simulink subsystem "cascaded_pid_controller_cgn"  (R2025b)
settings: Solver=VariableStepAuto  StartTime=0.0  StopTime=10.0  RelTol=1e-3
undefined symbols (not defined in the file or in its folder): allow_PID_resets_flag, const_voltage, DiscIntNeverNeededParam, do_force_cmd_flag, do_moment_cmd_flag, dRb_error_inject, dRb_PID, dRb_sp_inject, dspblkCoreblockFVToolHelper, dt_control, dt_data, Eul_e_tol, eul_error_inject, eul_sp_inject, FF_maneuvers, FT_list_inject, gcbh, invFT_wrench, invMT_wrench, overwrite_FT_list_flag, overwrite_rate_error_flag, overwrite_rate_setpoint_flag, overwrite_state_error_flag, overwrite_state_setpoint_flag, qib_PID, quat_pid_integrator_limit, Rb_error_inject, Rb_PID, Rb_sp_inject, Ri_e_tol, RSFF_maneuvers, wb_error_inject, wb_PID, wb_sp_inject
libraries: slpidlib x3, simulink x1
settings Model: Creator=vulcangrip  LastModifiedBy=vulcangrip

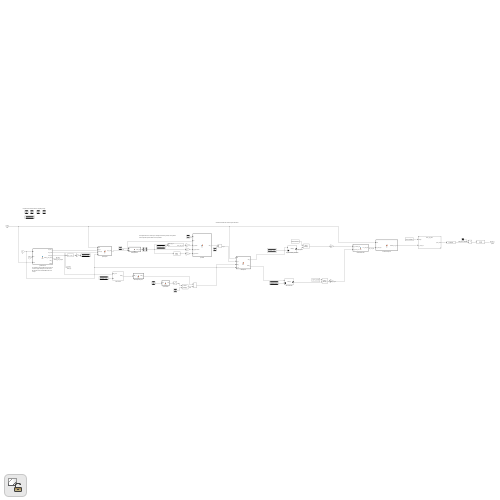
[thumbnail: Simulink's stored preview of the top-level diagram]
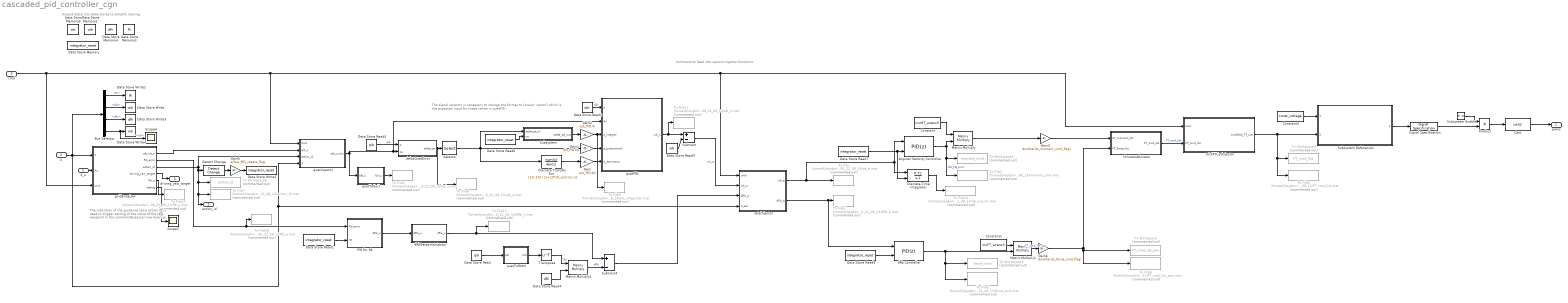
== system cascaded_pid_controller_cgn ==
  note: Unpack state into data-stores to simplify routing.
  note: Command to feed into various injector functions.
  note: The transition of the guidance law's action ID is used to trigger setting of the value of the idle waypoint in the commandExecuter one level up.
  note: The signal selector is necessary to change the format to [scalar; vector] which
      | is the expected input for these terms in quatPID.
  X_u : Inport  SampleTime=dt_control
  X : Inport  Port=2  SampleTime=dt_control
  cmd : Inport  Port=3  SampleTime=dt_control
  Subsystem Enable : EnablePort  PropagateVarSize=During execution  ShowOutputPort=on
  Angular Velocity Controller : slpidlib/PID Controller  Controller=PID  Form=Parallel  TimeDomain=Discrete-time  UseExternalTs=off  SampleTime=-1  IntegratorMethod=Forward Euler  FilterMethod=Forward Euler  ControllerParametersSource=internal  P=wb_PID.Kp  I=wb_PID.Ki  UseKiTs=off  D=wb_PID.Kd  UseExternalDerivativeSource=off  N=wb_PID.N  UseFilter=on  TunerSelectOption=Transfer Function Based (PID Tuner App)  InitialConditionSource=internal  InitialConditionForIntegrator=0  InitialConditionForFilter=0  DifferentiatorICPrevScaledInput=0  ExternalReset=rising  TrackingMode=off  Kt=1  LimitOutput=on  SatLimitsSource=internal  UpperSaturationLimit=wb_PID.output_sat  LowerSaturationLimit=-wb_PID.output_sat  LinearizeAsGain=on  AntiWindupMode=clamping  Kb=1  LimitIntegrator=on  UpperIntegratorSaturationLimit=wb_PID.int_sat  LowerIntegratorSaturationLimit=-wb_PID.int_sat  POutMin=[]  POutMax=[]  IOutMin=[]  IOutMax=[]  DOutMin=[]  DOutMax=[]  NOutMin=[]  NOutMax=[]  SumOutMin=[]  SumOutMax=[]  SaturationOutMin=[]  SaturationOutMax=[]  PParamMin=[]  PParamMax=[]  IParamMin=[]  IParamMax=[]  DParamMin=[]  DParamMax=[]  NParamMin=[]  NParamMax=[]  KbParamMin=[]  KbParamMax=[]  KtParamMin=[]  KtParamMax=[]  KbOutMin=[]  KbOutMax=[]  KtOutMin=[]  KtOutMax=[]  IntegratorOutMin=[]  IntegratorOutMax=[]  FilterOutMin=[]  FilterOutMax=[]  SumI1OutMin=[]  SumI1OutMax=[]  SumI2OutMin=[]  SumI2OutMax=[]  SumI3OutMin=[]  SumI3OutMax=[]  SumI4OutMin=[]  SumI4OutMax=[]  SumDOutMin=[]  SumDOutMax=[]  DifferentiatorOutMin=[]  DifferentiatorOutMax=[]  FilterDiffOutCoefMin=[]  FilterDiffOutCoefMax=[]  ReciprocalOutMin=[]  ReciprocalOutMax=[]  SumDenOutMin=[]  SumDenOutMax=[]  SumNumOutMin=[]  SumNumOutMax=[]  DivideOutMin=[]  DivideOutMax=[]  UdiffTsProdOutMin=[]  UdiffTsProdOutMax=[]  NTsProdOutMin=[]  NTsProdOutMax=[]  UintegralTsProdOutMin=[]  UintegralTsProdOutMax=[]  UngainTsProdOutMin=[]  UngainTsProdOutMax=[]  ClampingZeroOutDataTypeStr=Inherit: Inherit via back propagation  ClampingZeroOutMin=[]  ClampingZeroOutMax=[]  FilterDenConstantOutDataTypeStr=Inherit: Inherit via back propagation  FilterDenConstantOutMin=[]  FilterDenConstantOutMax=[]  PCopyOutDataTypeStr=Inherit: Inherit via back propagation  PCopyOutMin=[]  PCopyOutMax=[]  NCopyOutDataTypeStr=Inherit: Inherit via back propagation  NCopyOutMin=[]  NCopyOutMax=[]  IntegratorContinuousStateAttributes=''  IntegratorStateMustResolveToSignalObject=off  IntegratorRTWStateStorageClass=Auto  FilterContinuousStateAttributes=''  FilterStateMustResolveToSignalObject=off  FilterRTWStateStorageClass=Auto  ParallelPVariant=InternalParameters  IdealPVariant=Disabled  IVariant=InternalParameters  DVariant=InternalParameters  IntegratorVariant=Discrete  SatVariant=Enabled  AWVariant=DiscClampingParallel  PCopyVariant=Disabled  TRVariant=Disabled  FdbkBlocksVariant=Forward  IdealPFdbkVariant=Disabled  SatFdbkVariant=Disabled  DerivativeFilterVariant=ForwardEulerFilter  NVariant=InternalParameters  NCopyVariant=Disabled  FilterICVariant=InternalICsFilter  IntegratorICVariant=InternalICs  ExternalResetVariant=ExternalReset  TRSumVariant=Passthrough  SumFdbkVariant=Disabled  SumVariant=Sum_PID  TsampFilterVariant=InternalTs  TsampNgainVariant=Passthrough  TsampIntegralVariant=Disabled_SignalSpec  ExternalSaturationOutDataTypeStr=Inherit: Same as second input  DerivativeSourceVariant=ErrorSignal  PreIntVariant=InternalPreInt
  Bus Selector : BusSelector  OutputSignals=Ri,qib,dRi,wb
  Cast : DataTypeConversion  OutDataTypeStr=int32  SaturateOnIntegerOverflow=off  RndMeth=Floor
  Constant : Constant  Value=invMT_wrench
  Constant1 : Constant  Value=invFT_wrench
  Constant3 : Constant  Value=const_voltage
  Data Store Memory : DataStoreMemory  DataStoreName=integrator_reset  WriteAfterWriteMsg=warning  ShowAdditionalParam=off
  Data Store Memory2 : DataStoreMemory  DataStoreName=qib  WriteAfterWriteMsg=warning  InitialValue=[0 0 0 1]'  ShowAdditionalParam=off
  Data Store Memory3 : DataStoreMemory  DataStoreName=Ri  WriteAfterWriteMsg=warning  InitialValue=[0 0 0]'  ShowAdditionalParam=off
  Data Store Memory4 : DataStoreMemory  DataStoreName=dRi  WriteAfterWriteMsg=warning  InitialValue=[0 0 0]'  ShowAdditionalParam=off
  Data Store Memory5 : DataStoreMemory  DataStoreName=wb  WriteAfterWriteMsg=warning  InitialValue=[0 0 0]'  ShowAdditionalParam=off
  Data Store Read : DataStoreRead  DataStoreName=qib  IndexOptions=Index vector (dialog)  Indices=1  OutputSizes=1
  Data Store Read{1,6..7,9} (4 alike) : DataStoreRead  DataStoreName=integrator_reset  IndexOptions=Index vector (dialog)  Indices=1  OutputSizes=1
  Data Store Read2 : DataStoreRead  DataStoreName=qib  IndexOptions=Index vector (dialog)  Indices=1  OutputSizes=1
  Data Store Read3 : DataStoreRead  DataStoreName=wb  IndexOptions=Index vector (dialog)  Indices=1  OutputSizes=1
  Data Store Read4 : DataStoreRead  DataStoreName=dRi  IndexOptions=Index vector (dialog)  Indices=1  OutputSizes=1
  Data Store Read5 : DataStoreRead  DataStoreName=qib  IndexOptions=Index vector (dialog)  Indices=1  OutputSizes=1
  Data Store Write : DataStoreWrite  DataStoreName=qib  IndexOptions=Index vector (dialog)  Indices=1  OutputSizes=1
  Data Store Write1 : DataStoreWrite  DataStoreName=integrator_reset  IndexOptions=Index vector (dialog)  Indices=1  OutputSizes=1
  Data Store Write2 : DataStoreWrite  DataStoreName=Ri  IndexOptions=Index vector (dialog)  Indices=1  OutputSizes=1
  Data Store Write3 : DataStoreWrite  DataStoreName=dRi  IndexOptions=Index vector (dialog)  Indices=1  OutputSizes=1
  Data Store Write4 : DataStoreWrite  DataStoreName=wb  IndexOptions=Index vector (dialog)  Indices=1  OutputSizes=1
  Detect Change : simulink/Logic and Bit Operations/Detect Change  vinit=0  OutDataTypeStr=boolean
  Discrete Transfer Fcn : DiscreteTransferFcn  LoadFcn=dspblkCoreblockFVToolHelper(gcbh,'load');  Numerator=[10,-10]  Denominator=[1+10*dt_control,-1]
      settings: CopyFcn=dspblkCoreblockFVToolHelper(gcbh,'copy');  DeleteFcn=dspblkCoreblockFVToolHelper(gcbh,'close');  ModelCloseFcn=dspblkCoreblockFVToolHelper(gcbh,'close');  PreSaveFcn=dspblkCoreblockFVToolHelper(gcbh,'presave');  PostSaveFcn=dspblkCoreblockFVToolHelper(gcbh,'postsave');  CloseFcn=dspblkCoreblockFVToolHelper(gcbh,'close');
  Discrete-Time Integrator : DiscreteIntegrator  gainval=wb_PID.Ki  ExternalReset=rising  InitialCondition=[0;0;0]  SampleTime=dt_control  LimitOutput=on  UpperSaturationLimit=wb_PID.int_sat  LowerSaturationLimit=-wb_PID.int_sat  ICPrevOutput=DiscIntNeverNeededParam  ICPrevScaledInput=DiscIntNeverNeededParam
  Gain : Gain  Gain=qib_PID.Kd
  Gain1 : Gain  Gain=qib_PID.Kp
  Gain2 : Gain  Gain=qib_PID.Ki
  Gain3 : Gain  Gain=double(do_moment_cmd_flag)
  Gain4 : Gain  Gain=double(do_force_cmd_flag)
  Gain5 : Gain  Gain=allow_PID_resets_flag
  Matrix Multiply : Product  Multiplication=Matrix(*)
  Matrix Multiply1 : Product  Multiplication=Matrix(*)
  Matrix Multiply3 : Product  Multiplication=Matrix(*)
  PID for Rb : Subsystem
  Product : Product
  Scope1 : Scope
      settings: ActiveDisplayYMinimum=-1  ActiveDisplayYMaximum=1  DataLoggingVariableName=ScopeData3
  Scope4 : Scope
      settings: ActiveDisplayYMinimum=-1  ActiveDisplayYMaximum=1  DataLoggingVariableName=ScopeData6
  Selector : Selector  InputPortWidth=4  IndexOptions=Index vector (dialog)  Indices=[4 1 2 3]  OutputSizes=1
  Signal Specification : SignalSpecification  OutDataTypeStr=double
  Subsystem : Subsystem
  Subsystem Reference1 : Subsystem  ReferencedSubsystem=force_to_pwm
  Subtract : Sum  Inputs=+-
  Subtract4 : Sum  Inputs=+-
  To File : ToFile  Commented=on  Filename=/home/kjhaydon/Github/Robosub/SimulinkPlant/data/2026_07_06_22_08_13/wb_e.mat  MatrixName=wb_e  SaveFormat=Timeseries  SampleTime=dt_data
  To File1 : ToFile  Commented=on  Filename=/home/kjhaydon/Github/Robosub/SimulinkPlant/data/2026_07_06_22_08_13/dRb_e.mat  MatrixName=dRb_e  SaveFormat=Timeseries  SampleTime=dt_data
  To File10 : ToFile  Commented=on  Filename=/home/kjhaydon/Github/Robosub/SimulinkPlant/data/2026_07_06_22_08_13/Rb_e.mat  MatrixName=Rb_e  SaveFormat=Timeseries  SampleTime=dt_data
  To File11 : ToFile  Commented=on  Filename=/home/kjhaydon/Github/Robosub/SimulinkPlant/data/2026_07_06_22_08_13/wb_u.mat  MatrixName=wb_u  SaveFormat=Timeseries  SampleTime=dt_data
  To File12 : ToFile  Commented=on  Filename=/home/kjhaydon/Github/Robosub/SimulinkPlant/data/2026_07_06_22_08_13/dRb_u.mat  MatrixName=dRb_u  SaveFormat=Timeseries  SampleTime=dt_data
  To File13 : ToFile  Commented=on  Filename=/home/kjhaydon/Github/Robosub/SimulinkPlant/data/2026_07_06_22_08_13/Rb_u.mat  MatrixName=Rb_u  SaveFormat=Timeseries  SampleTime=dt_data
  To File14 : ToFile  Commented=on  Filename=/home/kjhaydon/Github/Robosub/SimulinkPlant/data/2026_07_06_22_08_13/wb_pid_int.mat  MatrixName=wb_pid_int  SaveFormat=Timeseries  SampleTime=dt_data
  To File2 : ToFile  Commented=on  Filename=/home/kjhaydon/Github/Robosub/SimulinkPlant/data/2026_07_06_22_08_13/moment_cmd.mat  MatrixName=moment_cmd  SaveFormat=Timeseries  SampleTime=dt_data
  To File3 : ToFile  Commented=on  Filename=/home/kjhaydon/Github/Robosub/SimulinkPlant/data/2026_07_06_22_08_13/Eul_u.mat  MatrixName=Eul_u  SaveFormat=Timeseries  SampleTime=dt_data
  To File4 : ToFile  Commented=on  Filename=/home/kjhaydon/Github/Robosub/SimulinkPlant/data/2026_07_06_22_08_13/FT_cmd_list.mat  MatrixName=FT_cmd_list  SaveFormat=Timeseries  SampleTime=dt_data
  To File5 : ToFile  Commented=on  Filename=/home/kjhaydon/Github/Robosub/SimulinkPlant/data/2026_07_06_22_08_13/force_cmd.mat  MatrixName=force_cmd  SaveFormat=Timeseries  SampleTime=dt_data
  To File6 : ToFile  Commented=on  Filename=/home/kjhaydon/Github/Robosub/SimulinkPlant/data/2026_07_06_22_08_13/FT_cmd_list_pos.mat  MatrixName=FT_cmd_list_pos  SaveFormat=Timeseries
  To File7 : ToFile  Commented=on  Filename=/home/kjhaydon/Github/Robosub/SimulinkPlant/data/2026_07_06_22_08_13/action_id.mat  MatrixName=action_id  SaveFormat=Timeseries  SampleTime=dt_control
  To File8 : ToFile  Commented=on  Filename=/home/kjhaydon/Github/Robosub/SimulinkPlant/data/2026_07_06_22_08_13/qib_e.mat  MatrixName=qib_e  SaveFormat=Timeseries  SampleTime=dt_data
  To File9 : ToFile  Commented=on  Filename=/home/kjhaydon/Github/Robosub/SimulinkPlant/data/2026_07_06_22_08_13/qib_integrator.mat  MatrixName=qib_integrator  SaveFormat=Timeseries  SampleTime=dt_data
  To Workspace : ToWorkspace  Commented=on  VariableName=FT_cmd_list_pos  SaveFormat=Timeseries  SampleTime=dt_data
  To Workspace2 : ToWorkspace  Commented=on  VariableName=FT_cmd_list  SaveFormat=Timeseries  SampleTime=dt_data
  To Workspace3 : ToWorkspace  Commented=on  VariableName=force_cmd  SaveFormat=Timeseries  SampleTime=dt_data
  To Workspace4 : ToWorkspace  Commented=on  VariableName=moment_cmd  SaveFormat=Timeseries  SampleTime=dt_data
  To Workspace5 : ToWorkspace  Commented=on  VariableName=action_id  SaveFormat=Timeseries  SampleTime=dt_control
  Transpose : Math  Operator=transpose
  dRb Controller : slpidlib/PID Controller  Controller=PID  Form=Parallel  TimeDomain=Discrete-time  UseExternalTs=off  SampleTime=-1  IntegratorMethod=Forward Euler  FilterMethod=Forward Euler  ControllerParametersSource=internal  P=dRb_PID.Kp  I=dRb_PID.Ki  UseKiTs=off  D=dRb_PID.Kd  UseExternalDerivativeSource=off  N=dRb_PID.N  UseFilter=on  TunerSelectOption=Transfer Function Based (PID Tuner App)  InitialConditionSource=internal  InitialConditionForIntegrator=0  InitialConditionForFilter=0  DifferentiatorICPrevScaledInput=0  ExternalReset=rising  TrackingMode=off  Kt=1  LimitOutput=on  SatLimitsSource=internal  UpperSaturationLimit=dRb_PID.output_sat  LowerSaturationLimit=-dRb_PID.output_sat  LinearizeAsGain=on  AntiWindupMode=clamping  Kb=1  LimitIntegrator=on  UpperIntegratorSaturationLimit=dRb_PID.int_sat  LowerIntegratorSaturationLimit=-dRb_PID.int_sat  POutMin=[]  POutMax=[]  IOutMin=[]  IOutMax=[]  DOutMin=[]  DOutMax=[]  NOutMin=[]  NOutMax=[]  SumOutMin=[]  SumOutMax=[]  SaturationOutMin=[]  SaturationOutMax=[]  PParamMin=[]  PParamMax=[]  IParamMin=[]  IParamMax=[]  DParamMin=[]  DParamMax=[]  NParamMin=[]  NParamMax=[]  KbParamMin=[]  KbParamMax=[]  KtParamMin=[]  KtParamMax=[]  KbOutMin=[]  KbOutMax=[]  KtOutMin=[]  KtOutMax=[]  IntegratorOutMin=[]  IntegratorOutMax=[]  FilterOutMin=[]  FilterOutMax=[]  SumI1OutMin=[]  SumI1OutMax=[]  SumI2OutMin=[]  SumI2OutMax=[]  SumI3OutMin=[]  SumI3OutMax=[]  SumI4OutMin=[]  SumI4OutMax=[]  SumDOutMin=[]  SumDOutMax=[]  DifferentiatorOutMin=[]  DifferentiatorOutMax=[]  FilterDiffOutCoefMin=[]  FilterDiffOutCoefMax=[]  ReciprocalOutMin=[]  ReciprocalOutMax=[]  SumDenOutMin=[]  SumDenOutMax=[]  SumNumOutMin=[]  SumNumOutMax=[]  DivideOutMin=[]  DivideOutMax=[]  UdiffTsProdOutMin=[]  UdiffTsProdOutMax=[]  NTsProdOutMin=[]  NTsProdOutMax=[]  UintegralTsProdOutMin=[]  UintegralTsProdOutMax=[]  UngainTsProdOutMin=[]  UngainTsProdOutMax=[]  ClampingZeroOutDataTypeStr=Inherit: Inherit via back propagation  ClampingZeroOutMin=[]  ClampingZeroOutMax=[]  FilterDenConstantOutDataTypeStr=Inherit: Inherit via back propagation  FilterDenConstantOutMin=[]  FilterDenConstantOutMax=[]  PCopyOutDataTypeStr=Inherit: Inherit via back propagation  PCopyOutMin=[]  PCopyOutMax=[]  NCopyOutDataTypeStr=Inherit: Inherit via back propagation  NCopyOutMin=[]  NCopyOutMax=[]  IntegratorContinuousStateAttributes=''  IntegratorStateMustResolveToSignalObject=off  IntegratorRTWStateStorageClass=Auto  FilterContinuousStateAttributes=''  FilterStateMustResolveToSignalObject=off  FilterRTWStateStorageClass=Auto  ParallelPVariant=InternalParameters  IdealPVariant=Disabled  IVariant=InternalParameters  DVariant=InternalParameters  IntegratorVariant=Discrete  SatVariant=Enabled  AWVariant=DiscClampingParallel  PCopyVariant=Disabled  TRVariant=Disabled  FdbkBlocksVariant=Forward  IdealPFdbkVariant=Disabled  SatFdbkVariant=Disabled  DerivativeFilterVariant=ForwardEulerFilter  NVariant=InternalParameters  NCopyVariant=Disabled  FilterICVariant=InternalICsFilter  IntegratorICVariant=InternalICs  ExternalResetVariant=ExternalReset  TRSumVariant=Passthrough  SumFdbkVariant=Disabled  SumVariant=Sum_PID  TsampFilterVariant=InternalTs  TsampNgainVariant=Passthrough  TsampIntegralVariant=Disabled_SignalSpec  ExternalSaturationOutDataTypeStr=Inherit: Same as second input  DerivativeSourceVariant=ErrorSignal  PreIntVariant=InternalPreInt
  dRbSetpointInjector : MATLAB Function  TreatAsAtomicUnit=on
  deltaQuatError : MATLAB Function  TreatAsAtomicUnit=on
  guidanceLaw : MATLAB Function  TreatAsAtomicUnit=on
  quatInjector : MATLAB Function  TreatAsAtomicUnit=on
  quatPID : MATLAB Function  TreatAsAtomicUnit=on
  quatToEul1 : MATLAB Function  TreatAsAtomicUnit=on
  quatToRotm : MATLAB Function  TreatAsAtomicUnit=on
  rateInjector : MATLAB Function  TreatAsAtomicUnit=on
  thrusterAllocator : MATLAB Function  TreatAsAtomicUnit=on
  trickFTListInjector : MATLAB Function  TreatAsAtomicUnit=on
  pwms : Outport
  action_id : Outport  Port=2
  driving_yaw_target : Outport  Port=3
  wires:
  Signal Specification/1 -> Product/2
  Matrix Multiply3/1 -> Subtract4/2  "dRb"
  Bus Selector/2 -> Data Store Write/1  "<qib>"
  X/1 -> quatInjector/4(X), rateInjector/4(X_est), guidanceLaw/1(X), Bus Selector/1
  Gain3/1 -> thrusterAllocator/1(FT_moment_list)
  rateInjector/1(wb_e) -> Angular Velocity Controller/1, Discrete-Time Integrator/1, To File/1
  Cast/1 -> pwms/1
  Detect Change/1 -> Gain5/1
  Angular Velocity Controller/1 -> To File2/1, To Workspace4/1, Matrix Multiply/2  "Mb_FB_cmd"
  Data Store Read3/1 -> Subtract/2
  Subtract/1 -> rateInjector/2("wb_e ")  "wb_e"
  Subsystem Enable/1 -> Product/1
  Data Store Read2/1 -> quatPID/1(q)  "qib"
  Gain2/1 -> quatPID/3(q_integral), To File9/1
  Data Store Read6/1 -> Subsystem/2(rst)
  dRb Controller/1 -> To Workspace3/1, To File5/1, Matrix Multiply1/2
  Data Store Read5/1 -> deltaQuatError/1(q)  "qib"
  Data Store Read9/1 -> dRb Controller/2
  quatInjector/1(qib_u_out) -> quatToEul1/1(qib_u), quatPID/2(qu), deltaQuatError/2(qu)
  guidanceLaw/6(debug) -> Scope1/1
  Constant1/1 -> Matrix Multiply1/1
  quatToEul1/1(Eul_u) -> To File3/1
  Gain4/1 -> To Workspace/1, To File6/1, thrusterAllocator/2(FT_force_list)
  guidanceLaw/5(Rb_u) -> To File13/1
  Subtract4/1 -> rateInjector/3("dRb_e ")
  guidanceLaw/4(driving_yaw_target) -> driving_yaw_target/1
  Data Store Read/1 -> quatToRotm/1(qib)
  Discrete-Time Integrator/1 -> To File14/1
  Discrete Transfer Fcn/1 -> Gain/1
  Gain/1 -> quatPID/5(q_derivative)
  PID for Rb/1(dRb_u) -> dRbSetpointInjector/1("dRb_u ")
  rateInjector/2(dRb_e) -> dRb Controller/1, To File1/1
  quatPID/1(wb_u) -> To File11/1, Subtract/1
  thrusterAllocator/1(FT_cmd_list) -> trickFTListInjector/2(FT_cmd_list)  "FT_cmd_list"
  Data Store Read1/1 -> PID for Rb/2(rst)
  Gain1/1 -> quatPID/4(q_proportional)
  Matrix Multiply1/1 -> Gain4/1  "FT_cmd_list_pos"
  Bus Selector/4 -> Data Store Write4/1, Scope4/1  "<wb>"
  guidanceLaw/3(action_id) -> quatInjector/3(action_id), action_id/1, To File7/1, To Workspace5/1, Detect Change/1
  X_u/1 -> guidanceLaw/2(Xu)
  Constant/1 -> Matrix Multiply/1
  Bus Selector/1 -> Data Store Write2/1  "<Ri>"
  dRbSetpointInjector/1(dRb_u) -> To File12/1, Subtract4/1
  Data Store Read7/1 -> Discrete-Time Integrator/2, Angular Velocity Controller/2
  Product/1 -> Cast/1
  Transpose/1 -> Matrix Multiply3/1  "Cbi"
  Gain5/1 -> Data Store Write1/1
  guidanceLaw/1(qib_int_u) -> quatInjector/2(qib_u)
  guidanceLaw/2(Rb_error) -> To File10/1, PID for Rb/1(Rb_error)
  cmd/1 -> guidanceLaw/3(cmd), trickFTListInjector/1(cmd), rateInjector/1(cmd), quatInjector/1(cmd)
  Constant3/1 -> Subsystem Reference1/1
  Subsystem Reference1/1 -> Signal Specification/1
  Matrix Multiply/1 -> Gain3/1
  Selector/1 -> Gain1/1, Discrete Transfer Fcn/1, Subsystem/1(delta_qe_in)
  Subsystem/1(delta_qe_out) -> Gain2/1
  trickFTListInjector/1(modified_FT_List) -> Subsystem Reference1/2, To File4/1, To Workspace2/1
  Bus Selector/3 -> Data Store Write3/1  "<dRi>"
  deltaQuatError/1(delta_qe) -> Selector/1, To File8/1
  Data Store Read4/1 -> Matrix Multiply3/2
  quatToRotm/1(Cib) -> Transpose/1

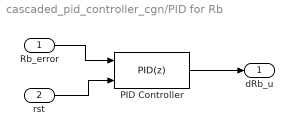
== system cascaded_pid_controller_cgn/PID for Rb ==
  Rb_error : Inport
  rst : Inport  Port=2
  PID Controller : slpidlib/PID Controller  Controller=PID  Form=Parallel  TimeDomain=Discrete-time  UseExternalTs=off  SampleTime=-1  IntegratorMethod=Forward Euler  FilterMethod=Forward Euler  ControllerParametersSource=internal  P=Rb_PID.Kp  I=Rb_PID.Ki  UseKiTs=off  D=Rb_PID.Kd  UseExternalDerivativeSource=off  N=Rb_PID.N  UseFilter=on  TunerSelectOption=Transfer Function Based (PID Tuner App)  InitialConditionSource=internal  InitialConditionForIntegrator=0  InitialConditionForFilter=0  DifferentiatorICPrevScaledInput=0  ExternalReset=rising  TrackingMode=off  Kt=1  LimitOutput=on  SatLimitsSource=internal  UpperSaturationLimit=Rb_PID.output_sat  LowerSaturationLimit=-Rb_PID.output_sat  LinearizeAsGain=on  AntiWindupMode=clamping  Kb=1  LimitIntegrator=on  UpperIntegratorSaturationLimit=Rb_PID.int_sat  LowerIntegratorSaturationLimit=-Rb_PID.int_sat  POutMin=[]  POutMax=[]  IOutMin=[]  IOutMax=[]  DOutMin=[]  DOutMax=[]  NOutMin=[]  NOutMax=[]  SumOutMin=[]  SumOutMax=[]  SaturationOutMin=[]  SaturationOutMax=[]  PParamMin=[]  PParamMax=[]  IParamMin=[]  IParamMax=[]  DParamMin=[]  DParamMax=[]  NParamMin=[]  NParamMax=[]  KbParamMin=[]  KbParamMax=[]  KtParamMin=[]  KtParamMax=[]  KbOutMin=[]  KbOutMax=[]  KtOutMin=[]  KtOutMax=[]  IntegratorOutMin=[]  IntegratorOutMax=[]  FilterOutMin=[]  FilterOutMax=[]  SumI1OutMin=[]  SumI1OutMax=[]  SumI2OutMin=[]  SumI2OutMax=[]  SumI3OutMin=[]  SumI3OutMax=[]  SumI4OutMin=[]  SumI4OutMax=[]  SumDOutMin=[]  SumDOutMax=[]  DifferentiatorOutMin=[]  DifferentiatorOutMax=[]  FilterDiffOutCoefMin=[]  FilterDiffOutCoefMax=[]  ReciprocalOutMin=[]  ReciprocalOutMax=[]  SumDenOutMin=[]  SumDenOutMax=[]  SumNumOutMin=[]  SumNumOutMax=[]  DivideOutMin=[]  DivideOutMax=[]  UdiffTsProdOutMin=[]  UdiffTsProdOutMax=[]  NTsProdOutMin=[]  NTsProdOutMax=[]  UintegralTsProdOutMin=[]  UintegralTsProdOutMax=[]  UngainTsProdOutMin=[]  UngainTsProdOutMax=[]  ClampingZeroOutDataTypeStr=Inherit: Inherit via back propagation  ClampingZeroOutMin=[]  ClampingZeroOutMax=[]  FilterDenConstantOutDataTypeStr=Inherit: Inherit via back propagation  FilterDenConstantOutMin=[]  FilterDenConstantOutMax=[]  PCopyOutDataTypeStr=Inherit: Inherit via back propagation  PCopyOutMin=[]  PCopyOutMax=[]  NCopyOutDataTypeStr=Inherit: Inherit via back propagation  NCopyOutMin=[]  NCopyOutMax=[]  IntegratorContinuousStateAttributes=''  IntegratorStateMustResolveToSignalObject=off  IntegratorRTWStateStorageClass=Auto  FilterContinuousStateAttributes=''  FilterStateMustResolveToSignalObject=off  FilterRTWStateStorageClass=Auto  ParallelPVariant=InternalParameters  IdealPVariant=Disabled  IVariant=InternalParameters  DVariant=InternalParameters  IntegratorVariant=Discrete  SatVariant=Enabled  AWVariant=DiscClampingParallel  PCopyVariant=Disabled  TRVariant=Disabled  FdbkBlocksVariant=Forward  IdealPFdbkVariant=Disabled  SatFdbkVariant=Disabled  DerivativeFilterVariant=ForwardEulerFilter  NVariant=InternalParameters  NCopyVariant=Disabled  FilterICVariant=InternalICsFilter  IntegratorICVariant=InternalICs  ExternalResetVariant=ExternalReset  TRSumVariant=Passthrough  SumFdbkVariant=Disabled  SumVariant=Sum_PID  TsampFilterVariant=InternalTs  TsampNgainVariant=Passthrough  TsampIntegralVariant=Disabled_SignalSpec  ExternalSaturationOutDataTypeStr=Inherit: Same as second input  DerivativeSourceVariant=ErrorSignal  PreIntVariant=InternalPreInt
  dRb_u : Outport
  wires:
  rst/1 -> PID Controller/2
  PID Controller/1 -> dRb_u/1
  Rb_error/1 -> PID Controller/1

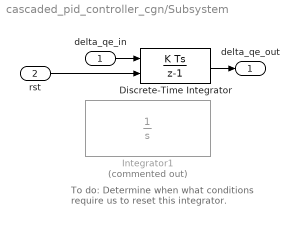
== system cascaded_pid_controller_cgn/Subsystem ==
  note: To do: Determine when what conditions
      | require us to reset this integrator.
  delta_qe_in : Inport
  rst : Inport  Port=2
  Discrete-Time Integrator : DiscreteIntegrator  ExternalReset=rising  SampleTime=-1  LimitOutput=on  UpperSaturationLimit=qib_PID.int_sat  LowerSaturationLimit=-qib_PID.int_sat  ICPrevOutput=DiscIntNeverNeededParam  ICPrevScaledInput=DiscIntNeverNeededParam
  Integrator1 : Integrator  Commented=on  ExternalReset=rising  LimitOutput=on  UpperSaturationLimit=quat_pid_integrator_limit  LowerSaturationLimit=-quat_pid_integrator_limit
  delta_qe_out : Outport
  wires:
  rst/1 -> Discrete-Time Integrator/2
  Discrete-Time Integrator/1 -> delta_qe_out/1
  delta_qe_in/1 -> Discrete-Time Integrator/1

== matlab function cascaded_pid_controller_cgn/quatToRotm ==
  data: qib input; Cib output
function Cib = fcn(qib)

Cib = quatToRotm(qib);

== matlab function cascaded_pid_controller_cgn/thrusterAllocator ==
  data: FT_moment_list input; FT_cmd_list output; FT_force_list input; max_thruster_force parameter
function FT_cmd_list = fcn(FT_moment_list, FT_force_list, max_thruster_force)

FT_cmd_list = thrusterAllocator(FT_moment_list, FT_force_list, max_thruster_force);

== matlab function cascaded_pid_controller_cgn/quatInjector ==
  data: cmd input; qib_u_out output; qib_u input; action_id input; X input; eul_sp_inject parameter; overwrite_state_setpoint_flag parameter
function qib_u_out  = fcn(cmd, qib_u, action_id, X, eul_sp_inject, overwrite_state_setpoint_flag)

qib_u_out = quatInjector(cmd, qib_u, action_id, X, eul_sp_inject, overwrite_state_setpoint_flag);

== matlab function cascaded_pid_controller_cgn/quatToEul1 ==
  data: qib_u input; Eul_u output
function Eul_u = fcn(qib_u)

Eul_u = quatToEul(qib_u);

== matlab function cascaded_pid_controller_cgn/dRbSetpointInjector ==
  data: dRb_u input; dRb_u output; overwrite_rate_setpoint_flag parameter; dRb_sp_inject parameter
function dRb_u=fcn(dRb_u, overwrite_rate_setpoint_flag, dRb_sp_inject)

if(overwrite_rate_setpoint_flag)
    dRb_u = dRb_sp_inject;
end

== matlab function cascaded_pid_controller_cgn/rateInjector ==
  data: cmd input Bus: cmd_bus; wb_e input; wb_e output; dRb_e input; dRb_e output; RSFF_maneuvers parameter Bus: RSFF_maneuver_bus; X_est input Bus: X_bus; overwrite_rate_error_flag parameter; wb_error_inject parameter; dRb_error_inject parameter
function [wb_e, dRb_e] = fcn(cmd, wb_e, dRb_e, RSFF_maneuvers, X_est, overwrite_rate_error_flag, wb_error_inject, dRb_error_inject)

[wb_e, dRb_e] = rateInjector(cmd, wb_e, dRb_e, X_est, RSFF_maneuvers, overwrite_rate_error_flag, wb_error_inject, dRb_error_inject);

== matlab function cascaded_pid_controller_cgn/trickFTListInjector ==
  data: cmd input; modified_FT_List output size=[8,1]; FT_cmd_list input; FF_maneuvers parameter Bus: FF_maneuvers_bus; overwrite_FT_list_flag parameter; FT_list_inject parameter size=[8,1]
function modified_FT_List = fcn(cmd, FT_cmd_list, FF_maneuvers, overwrite_FT_list_flag, FT_list_inject)

modified_FT_List = trickFTListInjector(cmd, FT_cmd_list, FF_maneuvers, overwrite_FT_list_flag, FT_list_inject);

== matlab function cascaded_pid_controller_cgn/guidanceLaw ==
  settings: updateMethod=DISCRETE  sampleTime=dt_control
  data: X input Bus: X_bus; qib_int_u output; Xu input; Rb_error output; Ri_e_tol parameter; action_id output; Eul_e_tol parameter; driving_yaw_target output; cmd input Bus: cmd_bus; Rb_u output; overwrite_state_error_flag parameter; Rb_error_inject parameter; overwrite_state_setpoint_flag parameter; Rb_sp_inject parameter; debug output
function [qib_int_u, Rb_error, action_id, driving_yaw_target, Rb_u,debug] = fcn(X, Xu, Ri_e_tol, Eul_e_tol, cmd, overwrite_state_error_flag, Rb_error_inject, overwrite_state_setpoint_flag, Rb_sp_inject)

[qib_int_u, Rb_error, action_id, driving_yaw_target, Rb_u,debug] = guidanceLaw(X, Xu, Ri_e_tol, Eul_e_tol, cmd, overwrite_state_error_flag, Rb_error_inject, overwrite_state_setpoint_flag, Rb_sp_inject);

== matlab function cascaded_pid_controller_cgn/deltaQuatError ==
  data: q input; delta_qe output; qu input; overwrite_state_error_flag parameter; eul_error_inject parameter
function delta_qe = fcn(q, qu, overwrite_state_error_flag, eul_error_inject)

delta_qe = deltaQuatError(q, qu, overwrite_state_error_flag, eul_error_inject);

== matlab function cascaded_pid_controller_cgn/quatPID ==
  data: q input; qu input; q_integral input; q_proportional input; wb_u output; q_derivative input; overwrite_rate_setpoint_flag parameter; wb_sp_inject parameter
function wb_u = fcn(q, qu, q_integral, q_proportional, q_derivative, overwrite_rate_setpoint_flag, wb_sp_inject)

wb_u = quatPID(q, qu, q_proportional, q_integral, q_derivative, overwrite_rate_setpoint_flag, wb_sp_inject);
